simulink model "blockdemo"  (Simulink 6.3)
settings: Solver=ode45  StartTime=0.0  StopTime=10.0  RelTol=1e-3
InitFcn:
  | %% DSPBuilder Start
  | alt_dspbuilder_update_model(bdroot)
  | %% DSPBuilder End
libraries: allblocks_alteradspbuilder2 x7
settings Model: Creator=cpurcell  LastModifiedBy=delphick
settings OptimizationCC: BooleanDataType=off  InlineInvariantSignals=on
settings DebuggingCC: SolverPrmCheckMsg=none
settings HardwareCC: TargetUnknown=on

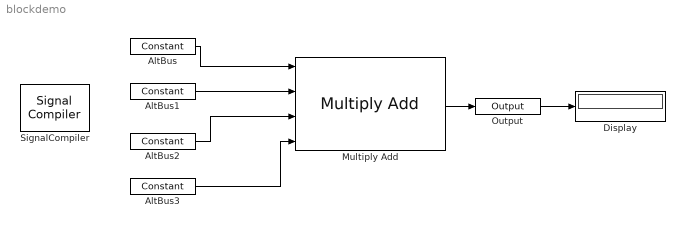
== system blockdemo ==
  AltBus{,1..3} (4 alike) : allblocks_alteradspbuilder2/Constant  mask_cst=5  BusType=Signed Integer  bwl=8  bwr=0  SpecifyClock=off
  Display : Display
  Multiply Add : allblocks_alteradspbuilder2/Multiply Add  multipliers=2  BusType=Signed Integer  bwl=8  bwr=0  direction=Sub Add  pipeline_register=Inputs Multiplier and Adder  use_constants=off  constants=[13 -2 0 3]  UseDedicatedCircuitry=off  use_ena=off  use_aclr=off
  Output : allblocks_alteradspbuilder2/Output  iofile=C:\workspace_clean\Documentation\DesignExamples\Tutorials\UnitBlocks\Arithmetic\MultiplyAdd\tb_blockdemo\blockdemo_Output.capture  BusType=Signed Integer  bwl=17  bwr=0  PORTTYPE=Output
  SignalCompiler : allblocks_alteradspbuilder2/Signal Compiler  DeviceFamily=Stratix IV  DeviceName=AUTO  EnableSignalTap=off  SignalTapDepth=128  UseBoardBlock=off  StpUseDefaultClock=on  StpClock=clock
  wires:
  Multiply Add/1 -> Output/1
  AltBus/1 -> Multiply Add/1
  AltBus1/1 -> Multiply Add/2
  AltBus2/1 -> Multiply Add/3
  AltBus3/1 -> Multiply Add/4
  Output/1 -> Display/1
